simulink model "model_quad_lqr_linear"  (R2021b)
settings: Solver=FixedStepAuto  StartTime=0.0  StopTime=10  FixedStep=.01  RelTol=1e-3
values from neighbouring files (symbols this model uses):
  A = reshape([mt1,mt2,mt3,mt4,mt5,mt6,mt7,mt8],12,12)    [Jacob.m]    (also in Lineared_SS_model.m = reshape([-1.097500e-06;0.000000e+00;0.000000e+00;-4.432200e-; find_optimal_lqr.m = reshape([-1.097500e-06;0.000000e+00;0.000000e+00;-4.432200e-; start_drone.m = zeros(12))
  B = reshape([mt9,mt10],12,4)    [Jacob.m]    (also in Lineared_SS_model.m = reshape([0.000000e+00;0.000000e+00;0.000000e+00;0.000000e+00; find_optimal_lqr.m = reshape([0.000000e+00;0.000000e+00;0.000000e+00;0.000000e+00; nlStateFcn.m = [0 0 0]; start_drone.m = zeros(12,4))
  K = reshape([-5.110766e+00;-5.110828e+00;5.110766e+00;5.110828e+00;-5.110828e+00;5.110766e+00;5.110828e+00;-5.110766e+00;-5.404988e+00;-5.404988e+00;-5.404988e+00;-5.404988e+00;-4.040006e+00;4.040001e+00;4.040006e+00;-4.040001e+00;4.040001e+00;4.040006e+00;-4.040001e+00;-4.040006e+00;-8.161851e-01;8.161851e-01;-8.161851e-01;8.161851e-01;-7.071059e+00;-7.071076e+00;7.071059e+00;7.071076e+00;-7.071076e+ ...(+481 chars)    [Lineared_SS_model.m]    (also in find_optimal_lqr.m = lqr(A,B,Q,R(i)); model_quad_init.m; start_drone.m = lqr(A,B,Q,R))
undefined symbols (not defined in the file or in its folder): Kdef
settings Model: Creator=Elena  LastModifiedBy=Elena

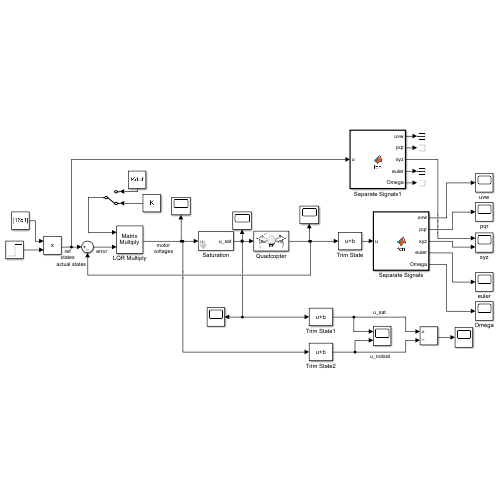
[thumbnail: Simulink's stored preview of the top-level diagram]
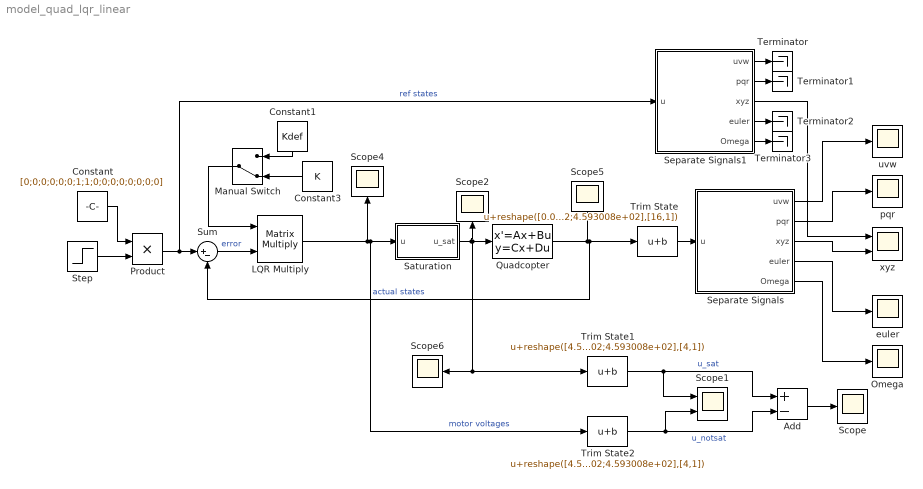
== system model_quad_lqr_linear ==
  Add : Sum  Inputs=+-
  Constant : Constant  Value=[0;0;0;0;0;0;1;1;0;0;0;0;0;0;0;0]
  Constant1 : Constant  Value=Kdef
  Constant3 : Constant  Value=K
  LQR Multiply : Product  Multiplication=Matrix(*)
  Manual Switch : ManualSwitch  CurrentSetting=0
  Omega : Scope
  Product : Product
  Quadcopter : StateSpace  A=A  B=B  C=eye(16)  D=zeros(16,4)  InitialCondition=0
      mask Display: image('drone_model.png'); % Use "Edit Image" on toolstrip to change.
  Saturation : Subsystem  mask{voltage_sat_upper=4*3.7-6.176, voltage_sat_lower=-6.176}
  Scope{,2,4..6} (5 alike) : Scope
  Scope1 : Scope  NumInputPorts=2
  Separate Signals : MATLAB Function  TreatAsAtomicUnit=on
  Separate Signals1 : MATLAB Function  TreatAsAtomicUnit=on
  Step : Step  After=2.2  SampleTime=0
  Sum : Sum  Inputs=|+-
  Terminator{,1..3} (4 alike) : Terminator
  Trim State : Bias  Bias=reshape([0.000000e+00;0.000000e+00;0.000000e+00;0.000000e+00;0.000000e+00;0.000000e+00;0.000000e+00;0.000000e+00;0.000000e+00;0.000000e+00;0.000000e+00;0.000000e+00;4.593008e+02;4.593008e+02;4.593008e+02;4.593008e+02],[16,1])
  Trim State1 : Bias  Bias=reshape([4.593008e+02;4.593008e+02;4.593008e+02;4.593008e+02],[4,1])
  Trim State2 : Bias  Bias=reshape([4.593008e+02;4.593008e+02;4.593008e+02;4.593008e+02],[4,1])
  euler : Scope
  pqr : Scope
  uvw : Scope
  xyz : Scope  NumInputPorts=2
  wires:
  Step/1 -> Product/2
  Quadcopter/1 -> Sum/2, Trim State/1, Scope5/1  "actual states"
  Constant/1 -> Product/1
  Product/1 -> Separate Signals1/1(u), Sum/1  "ref states"
  Separate Signals/3(xyz) -> xyz/2
  Separate Signals/2(pqr) -> pqr/1
  Separate Signals/1(uvw) -> uvw/1
  Separate Signals/4(euler) -> euler/1
  Separate Signals/5(Omega) -> Omega/1
  Sum/1 -> LQR Multiply/2  "error"
  Trim State/1 -> Separate Signals/1(u)
  Separate Signals1/3(xyz) -> xyz/1
  Separate Signals1/1(uvw) -> Terminator/1
  Separate Signals1/2(pqr) -> Terminator1/1
  Separate Signals1/4(euler) -> Terminator2/1
  Separate Signals1/5(Omega) -> Terminator3/1
  LQR Multiply/1 -> Trim State2/1, Saturation/1(u), Scope4/1  "motor voltages"
  Saturation/1(u_sat) -> Scope2/1, Scope6/1, Trim State1/1, Quadcopter/1
  Trim State1/1 -> Add/1, Scope1/1  "u_sat"
  Trim State2/1 -> Add/2, Scope1/2  "u_notsat"
  Add/1 -> Scope/1
  Constant3/1 -> Manual Switch/2
  Manual Switch/1 -> LQR Multiply/1
  Constant1/1 -> Manual Switch/1

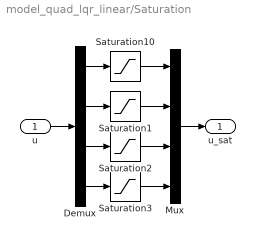
== system model_quad_lqr_linear/Saturation ==
  u : Inport
  Demux : Demux
  Mux : Mux
  Saturation{1..3,10} (4 alike) : Saturate  UpperLimit=voltage_sat_upper  LowerLimit=voltage_sat_lower
  u_sat : Outport
  wires:
  Demux/1 -> Saturation10/1
  Mux/1 -> u_sat/1
  Demux/2 -> Saturation1/1
  u/1 -> Demux/1
  Saturation10/1 -> Mux/1
  Saturation2/1 -> Mux/3
  Saturation1/1 -> Mux/2
  Saturation3/1 -> Mux/4
  Demux/3 -> Saturation2/1
  Demux/4 -> Saturation3/1

== matlab function model_quad_lqr_linear/Separate Signals1 ==
  data: u input; uvw output; pqr output; xyz output; euler output; Omega output
function [uvw,pqr,xyz,euler,Omega] = fcn(u)

uvw=u(1:3);
pqr=u((1:3)+3);
xyz=u((1:3)+6);
euler=u((1:3)+9);
Omega=u((1:4)+12);

== matlab function model_quad_lqr_linear/Separate Signals ==
  data: u input; uvw output; pqr output; xyz output; euler output; Omega output
function [uvw,pqr,xyz,euler,Omega] = fcn(u)

uvw=u(1:3);
pqr=u((1:3)+3);
xyz=u((1:3)+6);
euler=u((1:3)+9);
Omega=u((1:4)+12);
